simulink model "voicecoil"  (R2014a)
settings: Solver=ode3  StartTime=0.0  StopTime=40e-3  FixedStep=1e-7  RelTol=1e-3
undefined symbols (not defined in the file): L, Lambda_pm0oell, R
settings Model: CovSFcnEnable=on  Creator=Heath  LastModifiedBy=heath
settings DataIOCC: SignalLoggingSaveFormat=ModelDataLogs
settings OptimizationCC: ExpressionDepthLimit=2147483647
settings DebuggingCC: UnderspecifiedInitializationDetection=Classic  FcnCallInpInsideContextMsg=EnableAllAsWarning  FrameProcessingCompatibilityMsg=error  StateNameClashWarn=warning
settings GRTTargetCC: CombineOutputUpdateFcns=off  GRTInterface=on

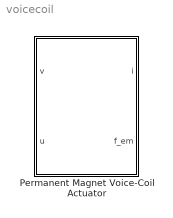
== system voicecoil ==
  Permanent Magnet Voice-Coil Actuator : Subsystem

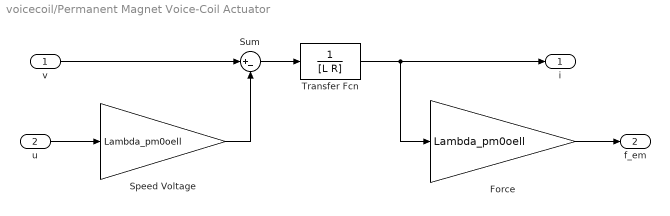
== system voicecoil/Permanent Magnet Voice-Coil Actuator ==
  v : Inport
  u : Inport  Port=2
  Force : Gain  Gain=Lambda_pm0oell
  Speed Voltage : Gain  Gain=Lambda_pm0oell
  Sum : Sum  Inputs=|+-
  Transfer Fcn : TransferFcn  Denominator=[L R]
  i : Outport
  f_em : Outport  Port=2
  wires:
  Transfer Fcn/1 -> i/1, Force/1
  Force/1 -> f_em/1
  v/1 -> Sum/1
  u/1 -> Speed Voltage/1
  Speed Voltage/1 -> Sum/2
  Sum/1 -> Transfer Fcn/1
